simulink model "user_io"  (Simulink 6.4)
settings: Solver=ode45  StartTime=0.0  StopTime=10.0  RelTol=1e-3
undefined symbols (not defined in the file): Down, Tsysclk, Up
libraries: xbsIndex_r4 x8, xrbsControl_r4 x2, xbsReplacements_r4 x2
settings Model: LastModifiedBy=docent

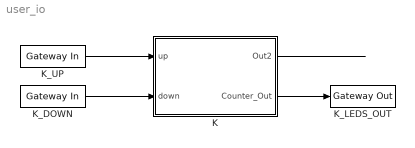
== system user_io ==
  K : Subsystem
  K_DOWN : xbsIndex_r4/Gateway In  arith_type=Boolean  n_bits=16  bin_pt=14  quantization="Round  (unbiased: +/- Inf)"  overflow=Saturate  period=Tsysclk*500  dbl_ovrd=off  timing_constraint=None  locs_specified=off  LOCs={}  block_type=gatewayin
      settings: infoedit="Gateway in block.  Converts inputs of type Simulink integer, double and fixed point to  Xilinx fixed point type.<P><P>Hardware notes:  In hardware these blocks become top level input ports."  xl_area=[0 0 0 0 16 0 0]  block_version=VER_STRING_GOES_HERE
  K_LEDS_OUT : xbsIndex_r4/Gateway Out  hdl_port=on  timing_constraint=None  locs_specified=off  LOCs={}  block_type=gatewayout
      settings: infoedit="Gateway out block.  Converts Xilinx fixed point inputs into ouputs of type Simulink integer, double, or fixed point.<P><P>Hardware notes:  In hardware these blocks become top level output ports or are discarded, depending on how they are configured."  xl_area=[0 0 0 0 16 0 0]  block_version=VER_STRING_GOES_HERE
  K_UP : xbsIndex_r4/Gateway In  arith_type=Boolean  n_bits=16  bin_pt=14  quantization="Round  (unbiased: +/- Inf)"  overflow=Saturate  period=Tsysclk*500  dbl_ovrd=off  timing_constraint=None  locs_specified=off  LOCs={}  block_type=gatewayin
      settings: infoedit="Gateway in block.  Converts inputs of type Simulink integer, double and fixed point to  Xilinx fixed point type.<P><P>Hardware notes:  In hardware these blocks become top level input ports."  xl_area=[0 0 0 0 16 0 0]  block_version=VER_STRING_GOES_HERE
  wires:
  K_UP/1 -> K/1(up)
  K/2(Counter_Out) -> K_LEDS_OUT/1
  K_DOWN/1 -> K/2(down)
  K/1(Out2) -> ?

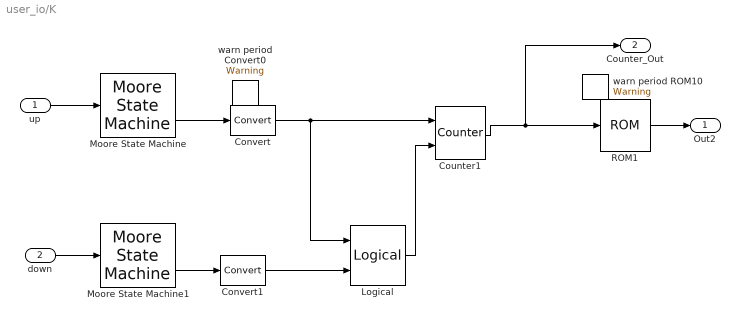
== system user_io/K ==
  up : Inport
  down : Inport  Port=2
  Convert : xbsIndex_r4/Convert  arith_type=Boolean  n_bits=8  bin_pt=6  quantization=Truncate  overflow=Wrap  latency=0  dbl_ovrd=off  pipeline=off  block_type=convert
      settings: xl_area=[0 0 0 0 0 0 0]  block_version=8.2.02
  Convert1 : xbsIndex_r4/Convert  arith_type=Boolean  n_bits=8  bin_pt=6  quantization=Truncate  overflow=Wrap  latency=0  dbl_ovrd=off  pipeline=off  block_type=convert
      settings: xl_area=[0 0 0 0 0 0 0]  block_version=8.2.02
  Counter1 : xbsIndex_r4/Counter  cnt_type=Free Running  cnt_to=Inf  operation=Up/Down  start_count=8  cnt_by_val=1  arith_type=Unsigned  n_bits=4  bin_pt=0  load_pin=off  rst=off  en=on  explicit_period=off  period=1  dbl_ovrd=off  use_behavioral_HDL=off  use_rpm=on  block_type=counter
      settings: xl_area=[2 4 0 4 0 0 0]  block_version=8.2.02
  Logical : xbsIndex_r4/Logical  logical_function=OR  inputs=2  en=off  latency=0  precision=Full  arith_type=Unsigned  n_bits=16  bin_pt=0  align_bp=on  dbl_ovrd=off  block_type=logical
      settings: block_version=8.2.02
  Moore State Machine : xrbsControl_r4/Moore State Machine  SystemSampleTime=-1  next_state_matrix=[0 1; 1 2; 0 2]  output_matrix=[0; 1; 0]  n_bits=1  period=1
  Moore State Machine1 : xrbsControl_r4/Moore State Machine  SystemSampleTime=-1  next_state_matrix=[0 1; 1 2; 0 2]  output_matrix=[0; 1; 0]  n_bits=1  period=1
  ROM1 : xbsIndex_r4/ROM  depth=16  initVector=(0.05:(0.95-0.05)/15:0.95)  distributed_mem=Block RAM  rst=off  init_reg=0  en=off  latency=1  arith_type="Signed  (2's comp)"  n_bits=16  bin_pt=14  dbl_ovrd=off  optimize=Area  use_rpm=off  block_type=sprom
      settings: xl_area=[0 0 1 0 0 0 0]  block_version=8.2.02
  warn period Convert0 : xbsReplacements_r4/Warning  SystemSampleTime=-1  period=1
  warn period ROM10 : xbsReplacements_r4/Warning  SystemSampleTime=-1  period=1
  Out2 : Outport
  Counter_Out : Outport  Port=2
  wires:
  Counter1/1 -> ROM1/1, Counter_Out/1
  Moore State Machine/2 -> Convert/1
  up/1 -> Moore State Machine/1
  ROM1/1 -> Out2/1
  Convert/1 -> Counter1/1, Logical/1
  down/1 -> Moore State Machine1/1
  Moore State Machine1/2 -> Convert1/1
  Logical/1 -> Counter1/2
  Convert1/1 -> Logical/2
